simulink model "P2_Ex8"  (R2021a)
settings: Solver=FixedStepAuto  StartTime=0.0  StopTime=Total_time  RelTol=1e-3
PreLoadFcn:
  | PreLoad_P2_Ex8
StopFcn:
  | post_P2_Ex8
values from neighbouring files (symbols this model uses):
  Ts = 0.01    [ejercicio8.m]
undefined symbols (not defined in the file or in its folder): Tg, Vmax
libraries: arduinolib x4
settings Model: SimulationMode=external  ExtModeTrigDuration=2  Creator=Eneko Lerma  LastModifiedBy=UPCnet
settings SolverCC: AlgebraicLoopSolver=TrustRegion
settings DataIOCC: ReturnWorkspaceOutputs=off
settings OptimizationCC: EnhancedBackFolding=on  PassReuseOutputArgsAs=Individual arguments  MaxStackSize=64  OptimizeBlockOrder=speed  DifferentSizesBufferReuse=on  OptimizationCustomize=off  EfficientTunableParamExpr=on
settings DebuggingCC: ParameterPrecisionLossMsg=none  ParameterTunabilityLossMsg=error  SFMachineParentedDataDiag=warning  ArithmeticOperatorsInVariantConditions=warning
settings HardwareCC: ProdBitPerPointer=32  ProdBitPerSizeT=32  ProdBitPerPtrDiffT=32  ProdLargestAtomicInteger=Long  ProdLargestAtomicFloat=Double  ProdWordSize=32  ProdHWDeviceType=ARM Compatible->ARM Cortex
settings SFSimCC: SimUseLocalCustomCode=off  MATLABDynamicMemAlloc=off  CustomCodeUndefinedFunction=UseInterfaceOnly
settings RTWCC: SystemTargetFile=ert.tlc  HardwareBoard=Arduino Due  TemplateMakefile=ert_default_tmf  GenerateReport=on  RTWUseLocalCustomCode=off  Toolchain=Arduino ARM  BuildConfiguration=Faster Runs  IncludeHyperlinkInReport=on  LaunchReport=on  GenerateTraceInfo=on  GenerateTraceReport=on  GenerateTraceReportSl=on  GenerateTraceReportSf=on  GenerateTraceReportEml=on
settings RTWCC: CustomTerminator=|
  | writeDigitalPin((uint8_T)3, 0);
  | writeDigitalPin((uint8_T)5, 0);
settings CodeAppCC: ForceParamTrailComments=on  IgnoreCustomStorageClasses=off  OperatorAnnotations=on  SimulinkDataObjDesc=on  SFDataObjDesc=on  InsertBlockDesc=on
settings ERTTargetCC: SupportContinuousTime=on  SupportVariableSizeSignals=on

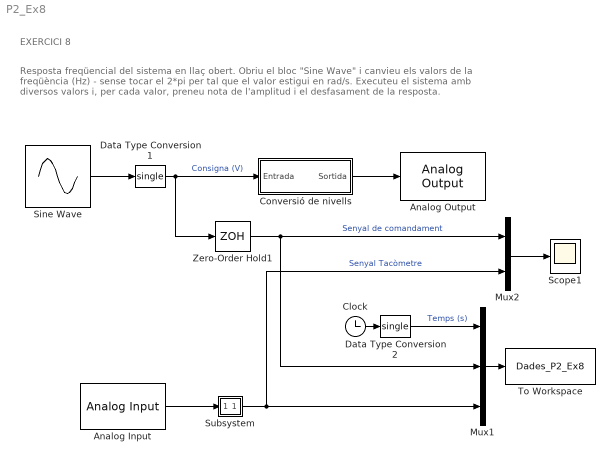
== system P2_Ex8 ==
  note: EXERCICI 8
  note: Resposta freqüencial del sistema en llaç obert. Obriu el bloc "Sine Wave" i canvieu els valors de la
      | freqüència (Hz) - sense tocar el 2*pi per tal que el valor estigui en rad/s. Executeu el sistema amb
      | diversos valors i, per cada valor, preneu nota de l'amplitud i el desfasament de la resposta.
  Analog Input : arduinolib/Analog Input  pinNumber=0  ReadResultsOnly=off  ConversionTriggerSource=Software  ExternalTriggerType=uint32(0)  OutputDataType=uint16  EnableConversionCompleteNotify=off  EnableOuputStatus=off  SampleTime=Tg  blockPlatform=arduino
  Analog Output : arduinolib/Analog Output  DACpin=DAC1  blockPlatform=arduino
      settings: SourceProductBaseCode=ARDUINO
  Clock : Clock
  Conversió de nivells : Subsystem
  Data Type Conversion1 : DataTypeConversion  OutDataTypeStr=single
  Data Type Conversion2 : DataTypeConversion  OutDataTypeStr=single
  Mux1 : Mux  Inputs=3
  Mux2 : Mux  Inputs=2
  Scope1 : Scope
  Sine Wave : Sin  Amplitude=Vmax  Frequency=2*pi*0.25  SampleTime=0
  Subsystem : Subsystem
  To Workspace : ToWorkspace  VariableName=Dades_P2_Ex8  SampleTime=-1
  Zero-Order Hold1 : ZeroOrderHold  SampleTime=Ts
  wires:
  Conversió de nivells/1(Sortida) -> Analog Output/1
  Sine Wave/1 -> Data Type Conversion1/1
  Clock/1 -> Data Type Conversion2/1
  Mux2/1 -> Scope1/1
  Data Type Conversion1/1 -> Conversió de nivells/1(Entrada), Zero-Order Hold1/1  "Consigna (V)"
  Mux1/1 -> To Workspace/1
  Data Type Conversion2/1 -> Mux1/1  "Temps (s)"
  Zero-Order Hold1/1 -> Mux2/1, Mux1/2  "Senyal de comandament"
  Subsystem/1("   ") -> Mux2/2, Mux1/3  "Senyal Tacòmetre"
  Analog Input/1 -> Subsystem/1(" ")

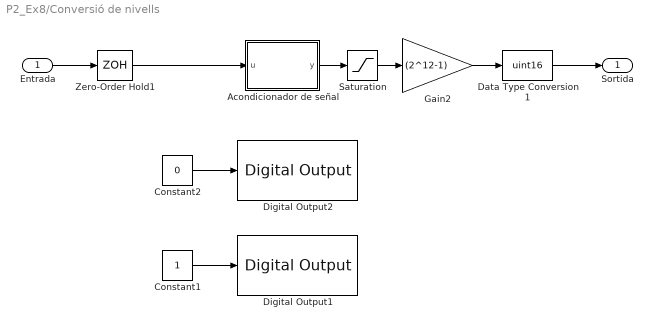
== system P2_Ex8/Conversió de nivells ==
  Entrada : Inport  OutDataTypeStr=single
  Acondicionador de señal : MATLAB Function  TreatAsAtomicUnit=on
  Constant1 : Constant
  Constant2 : Constant  Value=0
  Data Type Conversion1 : DataTypeConversion  OutDataTypeStr=uint16
  Digital Output1 : arduinolib/Digital Output  pinNumber=5  Direction=output  blockPlatform=arduino
  Digital Output2 : arduinolib/Digital Output  pinNumber=3  Direction=output  blockPlatform=arduino
  Gain2 : Gain  Gain=(2^12-1)  OutDataTypeStr=single
  Saturation : Saturate  UpperLimit=1  LowerLimit=0  OutDataTypeStr=single
  Zero-Order Hold1 : ZeroOrderHold  SampleTime=Ts
  Sortida : Outport  OutDataTypeStr=uint16  VectorParamsAs1DForOutWhenUnconnected=off
  wires:
  Saturation/1 -> Gain2/1
  Data Type Conversion1/1 -> Sortida/1
  Acondicionador de señal/1(y) -> Saturation/1
  Entrada/1 -> Zero-Order Hold1/1
  Gain2/1 -> Data Type Conversion1/1
  Zero-Order Hold1/1 -> Acondicionador de señal/1(u)
  Constant1/1 -> Digital Output1/1
  Constant2/1 -> Digital Output2/1

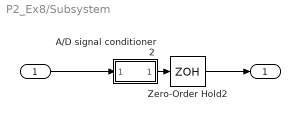
== system P2_Ex8/Subsystem ==
  " " : Inport
  A/D signal conditioner2 : Subsystem
  Zero-Order Hold2 : ZeroOrderHold  SampleTime=Ts
  "   " : Outport  VectorParamsAs1DForOutWhenUnconnected=off
  wires:
  A/D signal conditioner2/1(" ") -> Zero-Order Hold2/1
  Zero-Order Hold2/1 -> "   "/1
  " "/1 -> A/D signal conditioner2/1(" ")

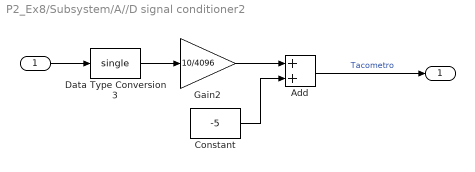
== system P2_Ex8/Subsystem/A//D signal conditioner2 ==
  " " : Inport
  Add : Sum  AccumDataTypeStr=single
  Constant : Constant  Value=-5  OutDataTypeStr=single
  Data Type Conversion3 : DataTypeConversion  OutDataTypeStr=single
  Gain2 : Gain  Gain=10/4096  OutDataTypeStr=single
  " " : Outport  VectorParamsAs1DForOutWhenUnconnected=off
  wires:
  " "/1 -> Data Type Conversion3/1
  Add/1 -> " "/1  "Tacometro"
  Gain2/1 -> Add/1
  Constant/1 -> Add/2
  Data Type Conversion3/1 -> Gain2/1

== matlab function P2_Ex8/Conversió de nivells/Acondicionador de señal ==
  data: u input; y output
function y = fcn(u)
y =0.0968*u+0.5058;
